simulink model "rpimulti_exec"  (Simulink 3.00)
libraries: execlib x12

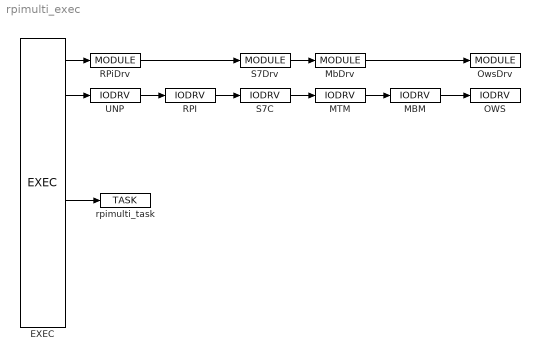
== system rpimulti_exec ==
  EXEC : execlib/EXEC  target=PC - Linux  tick=0.01  ntick0=2  ntick1=50  ntick2=100  ntick3=1200  pri0=5  pri1=9  pri2=13  pri3=18
  MBM : execlib/IODRV  module=MbDrv  classname=MbmDrv  cfgname=rpimulti_modbusRTUmaster.rio  factor=4  stack=10240  pri=3  timer=off
  MTM : execlib/IODRV  module=MbDrv  classname=MtmDrv  cfgname=rpimulti_modbusTCPmaster.rio  factor=2  stack=10240  pri=3  timer=off
  MbDrv : execlib/MODULE
  OWS : execlib/IODRV  module=OwsDrv  classname=OwsDrv  cfgname=rpimulti_1wire.rio  factor=50  stack=10240  pri=3  timer=off
  OwsDrv : execlib/MODULE
  RPI : execlib/IODRV  module=RPiDrv  classname=RPiDrv  factor=2  stack=10240  pri=3  timer=off
  RPiDrv : execlib/MODULE
  S7C : execlib/IODRV  module=S7Drv  classname=S7cDrv  cfgname=rpimulti_logo.rio  factor=2  stack=10240  pri=3  timer=off
  S7Drv : execlib/MODULE
  UNP : execlib/IODRV  module=RPiDrv  classname=UnpDrv  factor=2  stack=10240  pri=3  timer=off
  rpimulti_task : execlib/TASK  factor=1  start=0  stop=1  stack=10240  MDLOPEN=on
  wires:
  EXEC/1 -> RPiDrv/1
  EXEC/2 -> UNP/1
  EXEC/5 -> rpimulti_task/1
  MBM/1 -> OWS/1
  MTM/1 -> MBM/1
  MbDrv/1 -> OwsDrv/1
  RPI/1 -> S7C/1
  RPiDrv/1 -> S7Drv/1
  S7C/1 -> MTM/1
  S7Drv/1 -> MbDrv/1
  UNP/1 -> RPI/1
